simulink model "lab1"  (R2023a)
settings: Solver=VariableStepAuto  StartTime=0.0  StopTime=10.0  MaxStep=0.01  RelTol=1e-3
settings Model: Creator=Savely  LastModifiedBy=Admin

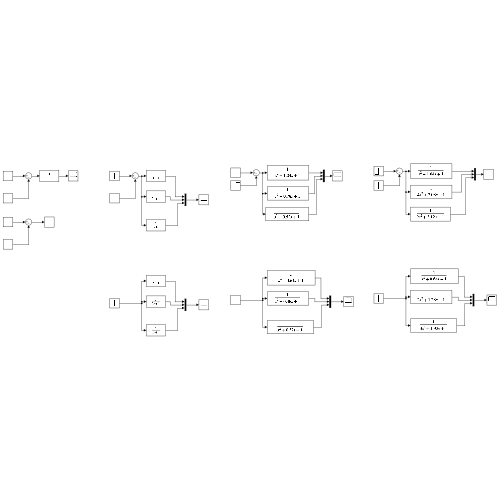
[thumbnail: Simulink's stored preview of the top-level diagram]
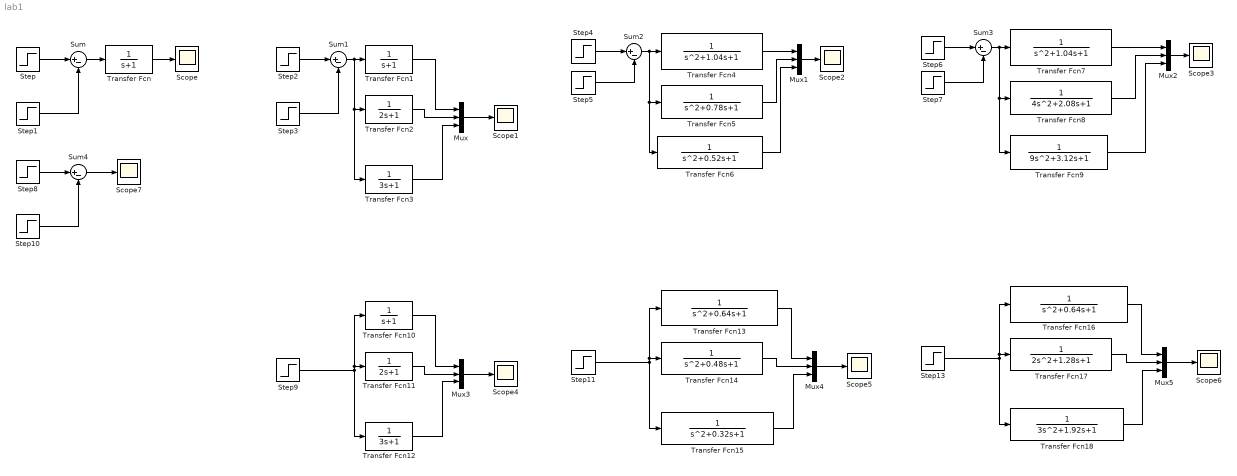
== system lab1 ==
  Mux{,1..5} (6 alike) : Mux  Inputs=3
  Scope{,1..7} (8 alike) : Scope
  Step{,2,4,6} (4 alike) : Step  Time=0  After=40  SampleTime=0
  Step1 : Step  Time=0.05  After=40  SampleTime=0
  Step10 : Step  SampleTime=0
  Step{3,5,7,9,11,13} (6 alike) : Step  Time=0.025  After=40  SampleTime=0
  Step8 : Step  Time=0  SampleTime=0
  Sum{,1..4} (5 alike) : Sum  Inputs=|+-
  Transfer Fcn : TransferFcn  Denominator=[1 1]
  Transfer Fcn1 : TransferFcn  Denominator=[1 1]
  Transfer Fcn10 : TransferFcn  Denominator=[1 1]
  Transfer Fcn11 : TransferFcn  Denominator=[2 1]
  Transfer Fcn12 : TransferFcn  Denominator=[3 1]
  Transfer Fcn13 : TransferFcn  Denominator=[1 0.64 1]
  Transfer Fcn14 : TransferFcn  Denominator=[1 0.48 1]
  Transfer Fcn15 : TransferFcn  Denominator=[1 0.32 1]
  Transfer Fcn16 : TransferFcn  Denominator=[1 0.64 1]
  Transfer Fcn17 : TransferFcn  Denominator=[2 1.28 1]
  Transfer Fcn18 : TransferFcn  Denominator=[3 1.92 1]
  Transfer Fcn2 : TransferFcn  Denominator=[2 1]
  Transfer Fcn3 : TransferFcn  Denominator=[3 1]
  Transfer Fcn4 : TransferFcn  Denominator=[1 1.04 1]
  Transfer Fcn5 : TransferFcn  Denominator=[1 0.78 1]
  Transfer Fcn6 : TransferFcn  Denominator=[1 0.52 1]
  Transfer Fcn7 : TransferFcn  Denominator=[1 1.04 1]
  Transfer Fcn8 : TransferFcn  Denominator=[4 2.08 1]
  Transfer Fcn9 : TransferFcn  Denominator=[9 3.12 1]
  wires:
  Step/1 -> Sum/1
  Step1/1 -> Sum/2
  Transfer Fcn/1 -> Scope/1
  Sum/1 -> Transfer Fcn/1
  Step2/1 -> Sum1/1
  Sum1/1 -> Transfer Fcn3/1, Transfer Fcn2/1, Transfer Fcn1/1
  Step3/1 -> Sum1/2
  Mux/1 -> Scope1/1
  Transfer Fcn1/1 -> Mux/1
  Transfer Fcn2/1 -> Mux/2
  Transfer Fcn3/1 -> Mux/3
  Transfer Fcn6/1 -> Mux1/3
  Transfer Fcn4/1 -> Mux1/1
  Sum2/1 -> Transfer Fcn6/1, Transfer Fcn5/1, Transfer Fcn4/1
  Transfer Fcn5/1 -> Mux1/2
  Step5/1 -> Sum2/2
  Mux1/1 -> Scope2/1
  Step4/1 -> Sum2/1
  Step6/1 -> Sum3/1
  Step7/1 -> Sum3/2
  Sum3/1 -> Transfer Fcn9/1, Transfer Fcn8/1, Transfer Fcn7/1
  Transfer Fcn7/1 -> Mux2/1
  Transfer Fcn8/1 -> Mux2/2
  Mux2/1 -> Scope3/1
  Transfer Fcn9/1 -> Mux2/3
  Transfer Fcn17/1 -> Mux5/2
  Transfer Fcn18/1 -> Mux5/3
  Transfer Fcn16/1 -> Mux5/1
  Step13/1 -> Transfer Fcn16/1, Transfer Fcn17/1, Transfer Fcn18/1
  Mux5/1 -> Scope6/1
  Step11/1 -> Transfer Fcn13/1, Transfer Fcn14/1, Transfer Fcn15/1
  Mux4/1 -> Scope5/1
  Transfer Fcn14/1 -> Mux4/2
  Transfer Fcn13/1 -> Mux4/1
  Transfer Fcn12/1 -> Mux3/3
  Transfer Fcn10/1 -> Mux3/1
  Step9/1 -> Transfer Fcn10/1, Transfer Fcn11/1, Transfer Fcn12/1
  Transfer Fcn15/1 -> Mux4/3
  Transfer Fcn11/1 -> Mux3/2
  Mux3/1 -> Scope4/1
  Sum4/1 -> Scope7/1
  Step10/1 -> Sum4/2
  Step8/1 -> Sum4/1
